simulink model "KD_cl_harness_forthao"  (R2015a)
settings: Solver=ode45  StartTime=0  StopTime=50  FixedStep=0.01  MaxStep=0.005  RelTol=1e-4  AbsTol=1e-4
InitFcn:
  | load KD_const_coeffs_0624
  | load pexhat_stuff
  | load expcon
  | load thr_ff_map
values from neighbouring files (symbols this model uses):
  c_0 = 0    [expcon.mat]
  c_1 = 1    [expcon.mat]
  c_100 = 100    [expcon.mat]
  c_1000 = 1000    [expcon.mat]
  c_10000 = 10000    [expcon.mat]
  c_1000inv = 0.0010000000475    [expcon.mat]    (also in pexhat_stuff.mat)
  c_100inv = 0.00999999977648    [expcon.mat]
  c_1_int = 1    [expcon.mat]
  c_1d2p4 = 0.416666656733    [expcon.mat]
  c_1p7 = 1.70000004768    [expcon.mat]
  c_4400inv = 0.000227272728807    [pexhat_stuff.mat]
  c_5500inv = 0.000181818177225    [expcon.mat]
  c_80 = 80    [expcon.mat]
  c_90 = 90    [expcon.mat]
  c_cal_phi = 7.6395999713e-06    [expcon.mat]
  c_compmap = [28125.0058594 29577.4082031 31350.1035156 33776.21875 37051.9296875 41026.2695312 45453.9960938 50160.3515625 55029.671875 59986.109375 64980.4296875 69980.4375 ... (320 elements, 20x16)]    [expcon.mat]
  c_ctok = 273.149993896    [expcon.mat]
  c_fflow_max = inf    [expcon.mat]
  c_fflow_min = 0    [expcon.mat]
  c_filt = 0.949999988079    [expcon.mat]
  c_flowdiv = 9.99999974738e-05    [expcon.mat]
  c_flowmin = 0    [expcon.mat]
  c_flowmult = 10000    [expcon.mat]
  c_inf = inf    [expcon.mat]
  c_km1d2k = 0.142857149243    [expcon.mat]
  c_mm3tokgpers = 2.77333338516e-08    [expcon.mat]
  c_n1 = -1    [expcon.mat]
  c_p00001 = 9.99999974738e-06    [expcon.mat]
  c_p01 = 0.00999999977648    [pexhat_stuff.mat]
  c_p016 = 0.01600000076    [expcon.mat]
  c_p1429 = 0.142900004983    [expcon.mat]
  c_p1e9 = 9.99999971718e-10    [expcon.mat]
  c_p4167 = 0.416700005531    [expcon.mat]    (also in pexhat_stuff.mat = 0.416666656733)
  c_p4d1p4 = 0.285714298487    [expcon.mat]
  c_p5401 = 0.540099978447    [expcon.mat]
  c_p9 = 0.899999976158    [expcon.mat]
  c_pincomp = 97.4216003418    [expcon.mat]
  c_ra = 287.002807617    [expcon.mat]
  c_rair = 287.09979248    [expcon.mat]
  c_Rby1000 = 0.000287000002572    [expcon.mat]
  c_roacorr = 8.05689978733e-06    [expcon.mat]
  c_rpmtoradpers = 0.104719758034    [expcon.mat]
  c_svrthrottle1 = [0.924875080585 0.575991511345 0.0858279466629 0.820202827454 0.445821881294 0.509882986546 0.0428557097912 0.753634572029 0]    [expcon.mat]
  c_svrthrottle2 = [0.145454958081 0.14545533061 0.363636374474 0.509091556072 0.509090721607 0.509091317654 0.545454084873 0.618182241917 0.145454272628]    [expcon.mat]
  c_svrthrottlearg = 0.10000000149    [expcon.mat]
  c_svrthrottlebeta = [2282.12670898 -3239.46044922 -142.784469604 -2660.34570312 1434.34350586 4150.43994141 -1580.68164062 -1039.89575195 791.34588623]    [expcon.mat]
  c_ta_max = inf    [expcon.mat]
  c_ta_min = 270    [expcon.mat]
  c_V = 0.0077999997884    [expcon.mat]
  c_vnliftmax = 90    [expcon.mat]
  c_vnliftmin = 40    [expcon.mat]
  Coefs =     [KD_const_coeffs_0624.mat]    (also in pexhat_stuff.mat)
  const =     [KD_const_coeffs_0624.mat]    (also in pexhat_stuff.mat)
  const_exhat =     [pexhat_stuff.mat]
  eegr_map =     [expcon.mat]
  egrr_delay_init = 0    [expcon.mat]
  epim_map =     [expcon.mat]
  eplufin_ff_map =     [expcon.mat]
  expcon =     [expcon.mat]
  invta = [5 5 5 5 2.5 0 0 0 0 0 0 0 ... (240 elements, 16x15)]    [expcon.mat]
  invtacols = [1000 1200 1400 1600 1800 2000 2200 2400 2600 2800 3000 3200 ... (16 elements, 1x16)]    [expcon.mat]
  IV =     [KD_const_coeffs_0624.mat]    (also in pexhat_stuff.mat)
  Lobs_init = [0 0 0]    [expcon.mat]
  map_delay_init = 120    [expcon.mat]
  maxA_t = [51.4567184448 53.8593139648 56.3063011169 58.7576789856 61.1701469421 63.4982337952 65.6955718994 67.7161483765 69.5156555176 71.0527648926 72.2902603149 73.1961746216 ... (16 elements, 1x16)]    [expcon.mat]
  obsA = [0.985195398331  0  0; -0.188821405172  1  0; 0.000342977960827  0  1]    [expcon.mat]
  sample_time = 0.016    [expcon.mat]    (also in pexhat_stuff.mat)
  SVR_EGR =     [KD_const_coeffs_0624.mat]    (also in pexhat_stuff.mat)
  SVR_EGR_exhat =     [pexhat_stuff.mat]
  SVR_throttle =     [KD_const_coeffs_0624.mat]    (also in pexhat_stuff.mat)
  uz_init = [0 0]    [expcon.mat]
undefined symbols (not defined in the file or in its folder): k1_table, k2_table, maxL, minL, Newton, Raphson
libraries: simulink x5
(part 6 of 6)

== system KD_cl_harness_forthao/ctrl_rb_explicit_20131031_v2/ntestimator/Throttle_Model/Air_Model_map_use/Forward_Flow/Cal_phi ==
  Ro_a : Inport
  Gain2 : Gain  Gain=c_roacorr  SaturateOnIntegerOverflow=on  OutDataTypeStr=Inherit: Same as input  ParamDataTypeStr=Inherit: Same as input
  Saturation : Saturate  UpperLimit=c_inf  LowerLimit=0
      settings: AttributesFormatString=%<LowerLimit>\n%<UpperLimit>
  Sqrt : Sqrt  AlgorithmType=Newton-Raphson  SaturateOnIntegerOverflow=on
  phi : Outport
  wires:
  Sqrt/1 -> phi/1
  Ro_a/1 -> Gain2/1
  Gain2/1 -> Saturation/1
  Saturation/1 -> Sqrt/1

== system KD_cl_harness_forthao/ctrl_rb_explicit_20131031_v2/ntestimator/Throttle_Model/Air_Model_map_use/Forward_Flow/For_Iterator_Subsystem ==
  u : Inport
  sv1 : Inport  Port=2
  sv2 : Inport  Port=3
  arg : Inport  Port=4
  beta : Inport  Port=5
  Demux : Demux  Outputs=2
  Divide : Product  Inputs=*/
  For Iterator : ForIterator  ResetStates=reset  IterationLimit=SVR_EGR_exhat.num_SV
  Gain : Gain  Gain=100
      settings: AttributesFormatString=%<Gain>
  Product{,1..3} (4 alike) : Product  RndMeth=Zero
  Saturation1 : Saturate  UpperLimit=9  LowerLimit=1
      settings: AttributesFormatString=%<LowerLimit>\n%<UpperLimit>
  Selector : Selector  InputPortWidth=SVR_EGR_exhat.num_SV  IndexOptions=Index vector (port)  Indices=[1 3]
  Selector1 : Selector  InputPortWidth=SVR_EGR_exhat.num_SV  IndexOptions=Index vector (port)  Indices=[1 3]
  Selector2 : Selector  InputPortWidth=SVR_EGR_exhat.num_SV  IndexOptions=Index vector (port)  Indices=[1 3]
  Sum : Sum  Inputs=|-+
  Sum1 : Sum  Inputs=+-|
  Sum2 : Sum  Inputs=-|-
  Sum3 : Sum  Inputs=++|
  Unit Delay : UnitDelay  SampleTime=-1
  exp Lookup Table : Lookup  InputValues=SVR_EGR_exhat.exp.x  Table=SVR_EGR_exhat.exp.y  LookUpMeth=Interpolation-Use End Values
      settings: AttributesFormatString=%<LookUpMeth>\n%<InputValues>
  ba : Outport  OutDataTypeStr=single
  wires:
  Saturation1/1 -> [iter]
  For Iterator/1 -> Saturation1/1
  [iter] -> Selector2/2
  [iter] -> Selector1/2
  [iter] -> Selector/2
  Sum3/1 -> ba/1, Unit Delay/1
  Product3/1 -> Sum3/2
  Selector2/1 -> Product3/2
  Gain/1 -> Divide/2
  Product2/1 -> Gain/1
  arg/1 -> Product2/2, Product2/1
  Sum2/1 -> Divide/1
  Product1/1 -> Sum2/2
  Product/1 -> Sum2/1
  Sum1/1 -> Product1/2, Product1/1
  Sum/1 -> Product/2, Product/1
  Demux/2 -> Sum1/1
  Selector1/1 -> Sum1/2
  Demux/1 -> Sum/2
  Selector/1 -> Sum/1
  u/1 -> Demux/1
  beta/1 -> Selector2/1
  sv2/1 -> Selector1/1
  sv1/1 -> Selector/1
  Unit Delay/1 -> Sum3/1
  Divide/1 -> exp Lookup Table/1
  exp Lookup Table/1 -> Product3/1

== matlab function KD_cl_harness_forthao/EGR Valve/SVR EGR/EGR_model/Air Model_map_use/Forward-Flow/SVR_EGR ==
  data: u input; B_A_spd output; num_SV input; Beta input; SV input; arg input
function B_A_spd = fcn(u, num_SV, Beta, SV, arg)
%#eml
Kern=zeros(length(SV),1);
    for n=1:num_SV
        v = SV(n,:).';
        Kern(n)=exp(-(u-v)'*(u-v)/(50*(2*arg^2)));
    end
B_A_spd = Beta.'*Kern;

== matlab function KD_cl_harness_forthao/Turbine/TurbineMap/TurbineMAP1 ==
  data: turb_pres_ratio input; omega_turbo input; p_in_turb input; T_ambient input; T_exh_man input; VNlift input; W_turbine_sim output; Turb_Constants input; TurbFlowCoefs input; TurbTempCoefs input; T_out_turbine output; eta_turb output; A_turbine output; phi output; delta_T_Turbo output; Tq_turbine output
 function [W_turbine_sim, T_out_turbine,eta_turb,A_turbine,phi,delta_T_Turbo,Tq_turbine] = TurbineMap(turb_pres_ratio,omega_turbo,p_in_turb,T_ambient,T_exh_man,VNlift,Turb_Constants, TurbFlowCoefs, TurbTempCoefs)

%% Reference: Turbocharger modelling for Automotive Control Applications by Paul Moraal and Ilya Kolmanovsky
% if T_exh_man <= 0
%     a = 1;
% end
Dia_turb = Turb_Constants(1); %Turbine diameter
Cp = Turb_Constants(2);  % Cp_Air_300K_KJ_per_kg_K
gamma_air = Turb_Constants(3);
eng_Vol = Turb_Constants(4);

PR= turb_pres_ratio;

%% putting saturartions on the blocks
PR = median([0.0001 PR 0.97]); % to avoid Zero-crossing errors

A_turbine  =   TurbFlowCoefs(1) +TurbFlowCoefs(2)*VNlift + TurbFlowCoefs(3)*omega_turbo +TurbFlowCoefs(4)*VNlift.^2 + TurbFlowCoefs(5)*omega_turbo.^2;

p_crit = ((gamma_air + 1)/2)^(gamma_air/(1 -gamma_air));

if PR > p_crit 
    phi_by_At = sqrt(((2*gamma_air)/(gamma_air-1))*(PR^(2/gamma_air) - PR^((gamma_air+1)/gamma_air)));
else
    phi_by_At = 0.6847;  %% check this value
end

phi = phi_by_At * A_turbine ;
phi = median([0.00001 phi 0.2]);
%%
%% to eliminate Zero crossing errors of  simulink
p_in_turb =  median([50 p_in_turb 1000]);
T_exh_man =  median([100 T_exh_man 2000]);

%%
W_turbine_sim = (phi * p_in_turb)/sqrt(T_exh_man); % kgpersec

U_by_C_den = 60*sqrt(2*Cp*T_exh_man*(1- (PR)^((gamma_air-1)/gamma_air)));

U_by_C = (pi* Dia_turb* omega_turbo)/U_by_C_den ;


delta_T_Turbo =  TurbTempCoefs(1) + TurbTempCoefs(2)*U_by_C +TurbTempCoefs(3)*PR...
    + TurbTempCoefs(4)*VNlift +TurbTempCoefs(5)*U_by_C^2 +  TurbTempCoefs(6)*PR^2 +TurbTempCoefs(7)*VNlift^2  ;

% delta_T_Turbo = median([ 0 delta_T_Turbo  250]);
T_out_turbine = T_exh_man - delta_T_Turbo;

eta_turb_num  = 1- (T_out_turbine/T_exh_man);
eta_turb_den = 1 - PR^(0.2857);
eta_turb = eta_turb_num/eta_turb_den ;

% Tq_in Newton meter
% %  Tq in N_m
Tq_turbine = (Cp*W_turbine_sim*delta_T_Turbo*60)/(2*pi*omega_turbo);

== matlab function KD_cl_harness_forthao/Intercooler/Intercooler/MATLAB Function ==
  data: T_in_IC input; T_ambient input; T_out_IC output; ICTempCoefs input
function T_out_IC = InterCoolerMap(T_in_IC,T_ambient,ICTempCoefs)
%#codegen

delT = T_in_IC - T_ambient;
T_out_IC= ICTempCoefs(1)*delT ^2+ ICTempCoefs(2)*delT + ICTempCoefs(3);

== matlab function KD_cl_harness_forthao/Compressor/Comp Map/MATLAB Function ==
  data: pres_Rat input; W_comp output; T_in_comp input; omega_turbo_RPM input; Comp_Constants input; CompPresRatCoefs input; CompEffCoefs input; T_out_comp output; P_comp_W output; pres_Rat1 output; Uc output; Mach output; psi output; k1 output; k2 output; k3 output; PhiC output; Comp_Efficiency output; PhiC1 output; a1 output; a2 output; a3 output; Tq_Compressor output
function [W_comp, T_out_comp,P_comp_W, pres_Rat1,Uc,Mach,psi,k1,k2,k3,PhiC,Comp_Efficiency,PhiC1,a1,a2,a3,Tq_Compressor]   = CompMap(pres_Rat,T_in_comp,omega_turbo_RPM,Comp_Constants,CompPresRatCoefs,CompEffCoefs)

%% Reference: Turbocharger modelling for Automotive Control Applications by Paul Moraal and Ilya Kolmanovsky

dc = Comp_Constants(1); % Compressor Diameter(Outer impeller diameter)
gamma_air = Comp_Constants(2);
R_air = Comp_Constants(3);   % R_specific_air_J_per_kg_kelvin
Cp_Air = Comp_Constants(4);  % Cp_Air_300K_J_per_kg_K
Rho_Air = Comp_Constants(5); % rho_Air_300K_kg_per_m3

x_low = CompPresRatCoefs(1:6);
x_high = CompPresRatCoefs(7:12);

Ntc_cutoff = 25000;
ratio = 0.5*(1 + tanh(((omega_turbo_RPM-Ntc_cutoff)*2*pi)/Ntc_cutoff));
PRcoeffs = (1-ratio)*x_low + ratio*x_high;

% pres_Rat = p_out_comp/p_in_comp;

pres_Rat1 = pres_Rat;
% pres_Rat = median([1 pres_Rat 3]);
% limit pressure ratio accordingly

%% Uc  = Blade speed
Uc = (pi/60)*dc*omega_turbo_RPM;  %% Equation 24

%% Mach = Mach Number
Mach = Uc/(sqrt(gamma_air*R_air*T_in_comp));  %% Equation 26

%% psi = slip factor
psi_num = Cp_Air*T_in_comp*((pres_Rat^((gamma_air -1)/gamma_air))-1);
psi_den = 0.5*Uc*Uc;
psi = psi_num/psi_den;   %% head parameter Equation 23
psi = median([0.0003 psi 10]);

k1 = PRcoeffs(1) + PRcoeffs(2)*Mach;
k2 = PRcoeffs(3) + PRcoeffs(4)*Mach;
k3 = PRcoeffs(5) + PRcoeffs(6)*Mach;

PhiC = ((k3*psi)-k1)/(k2+psi); %%Normalized compressor flow %% Equation 29
PhiC1 = PhiC;
W_comp = PhiC*Rho_Air*(pi/4)*dc*dc*Uc;
W_comp = median([0.0010 W_comp 0.3]);

% % Efficency Calculations

a1 = (CompEffCoefs(1) +  CompEffCoefs(2)*Mach)/(CompEffCoefs(3) - Mach);
a2 = (CompEffCoefs(4) +  CompEffCoefs(5)*Mach)/(CompEffCoefs(6) - Mach);
a3 = (CompEffCoefs(7) +  CompEffCoefs(8)*Mach)/(CompEffCoefs(9) - Mach);

% A = [a1 a2 a3];
Comp_Efficiency = a1*PhiC^2 + a2*PhiC + a3; %%Equation 27
% Comp_Efficiency = median([0.01 Comp_Efficiency 1]);


delta_T_comp = (T_in_comp/Comp_Efficiency)*(pres_Rat^((gamma_air -1)/gamma_air) - 1);
delta_T_comp = median([7  delta_T_comp 150]);

T_out_comp = T_in_comp + delta_T_comp ;  %%Equation 5

P_comp_W = W_comp*Cp_Air*delta_T_comp ; %% power in KW

%% Tq in N-m
Tq_Compressor = (Cp_Air*W_comp*delta_T_comp*60)/(2*pi*omega_turbo_RPM) ;

== matlab function KD_cl_harness_forthao/EGR cooler/EGR Cooler/MATLAB Function ==
  data: T_in_EGR_cooler input; T_out_EGR_cooler output; T_coolant input; W_egr_valve input; EGRbypassflag input; engine_speed_RPM input; EGRCoolerTempCoefs input; EGRCoolerbypassTempCoefs input
function T_out_EGR_cooler   = EGRCoolerMap(T_in_EGR_cooler,T_coolant,W_egr_valve,EGRbypassflag,engine_speed_RPM, EGRCoolerTempCoefs,EGRCoolerbypassTempCoefs )
%#codegen

if EGRbypassflag > 1.5
    
    CoolerPercentEff =  EGRCoolerTempCoefs(1) + EGRCoolerTempCoefs(2)*T_in_EGR_cooler +EGRCoolerTempCoefs(3)*W_egr_valve  +EGRCoolerTempCoefs(4)*engine_speed_RPM...
                    +EGRCoolerTempCoefs(5)*T_in_EGR_cooler^2 + EGRCoolerTempCoefs(6)*W_egr_valve^2 + EGRCoolerTempCoefs(7)*engine_speed_RPM^2;
    
    T_out_EGR_cooler = T_in_EGR_cooler + (T_coolant - T_in_EGR_cooler)*CoolerPercentEff/100;
    
else
    T_out_EGR_cooler = EGRCoolerbypassTempCoefs(1) + EGRCoolerbypassTempCoefs(2)*T_in_EGR_cooler;

end

== matlab function KD_cl_harness_forthao/EGR Throttle/EGR Throttle/Throttle Model2/Air Model_map_use/Back-Flow/SVR_throttle ==
  data: u input; B_A_spd output; num_SV input; Beta input; SV input; arg input
function B_A_spd = fcn(u, num_SV, Beta, SV, arg)
%#eml
Kern=zeros(length(SV),1);
    for n=1:num_SV
        v = SV(n,:).';
        Kern(n)=exp(-(u-v)'*(u-v)/(50*(2*arg^2)));
    end
B_A_spd = Beta.'*Kern;

== matlab function KD_cl_harness_forthao/EGR Valve/SVR EGR/EGR_model/Air Model_map_use/Back-Flow/SVR_EGR ==
  data: u input; B_A_spd output; num_SV input; Beta input; SV input; arg input
function B_A_spd = fcn(u, num_SV, Beta, SV, arg)
%#eml
Kern=zeros(length(SV),1);
    for n=1:num_SV
        v = SV(n,:).';
        Kern(n)=exp(-(u-v)'*(u-v)/(50*(2*arg^2)));
    end
B_A_spd = Beta.'*Kern;

== matlab function KD_cl_harness_forthao/EGR Throttle/EGR Throttle/Throttle Model2/Air Model_map_use/Forward-Flow/SVR_throttle ==
  data: u input; B_A_spd output; num_SV input; Beta input; SV input; arg input
function B_A_spd = fcn(u, num_SV, Beta, SV, arg)
%#eml
Kern=zeros(length(SV),1);
    for n=1:num_SV
        v = SV(n,:).';
        Kern(n)=exp(-(u-v)'*(u-v)/(50*(2*arg^2)));
    end
B_A_spd = Beta.'*Kern;

== matlab function KD_cl_harness_forthao/Combsution/cylinder comp/MATLAB Function ==
  data: W_cyl_out output; omega_engine input; p_in_man input; p_exh_man input; T_in_man input; T_exh_man input; CylConstants input; cylFlowCoefs input; nVol output
function [W_cyl_out,nVol ]= CylinderMap(omega_engine, p_in_man,p_exh_man, T_in_man, T_exh_man,CylConstants,cylFlowCoefs)
%#codegen
% p_in_man
%% check this

%%constraints

T_exh_man =  median([100 T_exh_man 2000]);

cfs = cylFlowCoefs;
nVol = cfs(1) + cfs(2)*omega_engine + cfs(3)*omega_engine^2  + cfs(4)*p_exh_man + cfs(5)*p_in_man + cfs(6)*p_exh_man/sqrt(T_exh_man);   

W_cyl_out = (nVol * p_in_man *omega_engine *CylConstants(1))/(120*CylConstants(2) *T_in_man);

== matlab function KD_cl_harness_forthao/Combsution/Exhaust /MATLAB Function1 ==
  data: omega_engine_rpm input; T_exhaust output; T_in_man input; W_cyl input; u_fuel input; F1_in input; ExhaustTempCoefs input
function T_exhaust    = ExhaustTemp(omega_engine_rpm, T_in_man, W_cyl ,u_fuel, F1_in, ExhaustTempCoefs)
%#codegen

% based on previous engine model fit
% %  no data for doing estimation.
fuelFrac = u_fuel/(W_cyl + u_fuel);
T_exhaust = T_in_man + (ExhaustTempCoefs(1)+ExhaustTempCoefs(2)*fuelFrac +ExhaustTempCoefs(3)*omega_engine_rpm*fuelFrac + ExhaustTempCoefs(4)*F1_in);
